simulink model "geothermal_simulink"  (R2024a)
settings: Solver=VariableStepAuto  StartTime=0.0  StopTime=10.0  RelTol=1e-3
libraries: spsStairGeneratorLib x1
settings Model: Creator=dogba  LastModifiedBy=dogba

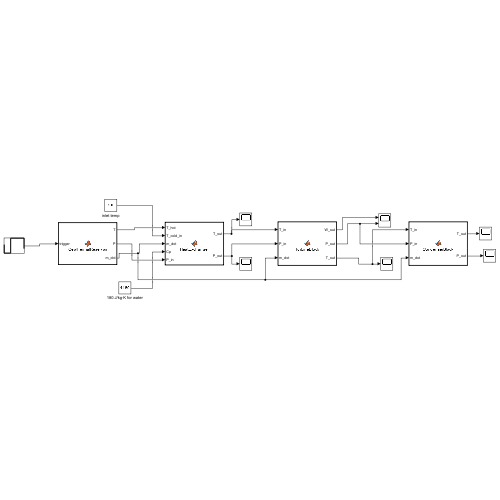
[thumbnail: Simulink's stored preview of the top-level diagram]
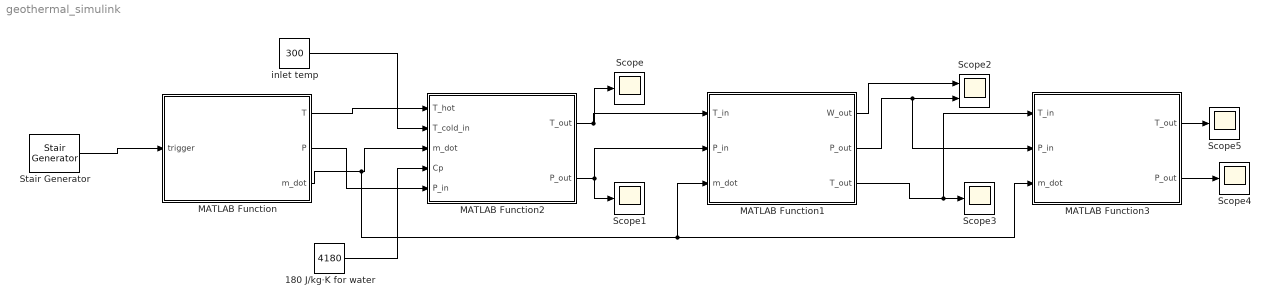
== system geothermal_simulink ==
  180 J/kg·K for water : Constant  Value=4180
  MATLAB Function : MATLAB Function  TreatAsAtomicUnit=on
  MATLAB Function1 : MATLAB Function  TreatAsAtomicUnit=on
  MATLAB Function2 : MATLAB Function  TreatAsAtomicUnit=on
  MATLAB Function3 : MATLAB Function  TreatAsAtomicUnit=on
  Scope{,1,3..5} (5 alike) : Scope
  Scope2 : Scope  NumInputPorts=2
  Stair Generator : spsStairGeneratorLib/Stair Generator  t=[0, 2,4, 8]  e=[1, -1, 2.5, 0]  Ts=0
  inlet temp : Constant  Value=300
  wires:
  MATLAB Function/2(P) -> MATLAB Function2/5(P_in)
  MATLAB Function/3(m_dot) -> MATLAB Function3/3(m_dot), MATLAB Function1/3(m_dot), MATLAB Function2/3(m_dot)
  MATLAB Function/1(T) -> MATLAB Function2/1(T_hot)
  180 J/kg·K for water/1 -> MATLAB Function2/4(Cp)
  inlet temp/1 -> MATLAB Function2/2(T_cold_in)
  MATLAB Function2/1(T_out) -> MATLAB Function1/1(T_in), Scope/1
  MATLAB Function2/2(P_out) -> Scope1/1, MATLAB Function1/2(P_in)
  MATLAB Function1/1(W_out) -> Scope2/1
  MATLAB Function1/2(P_out) -> MATLAB Function3/2(P_in), Scope2/2
  MATLAB Function1/3(T_out) -> MATLAB Function3/1(T_in), Scope3/1
  MATLAB Function3/2(P_out) -> Scope4/1
  MATLAB Function3/1(T_out) -> Scope5/1
  Stair Generator/1 -> MATLAB Function/1(trigger)

== matlab function geothermal_simulink/MATLAB Function1 ==
  data: W_out output; P_out output; T_in input; P_in input; T_out output; m_dot input
function [W_out, P_out, T_out] = TurbineBlock(T_in, P_in, m_dot)
% Custom turbine block
% Inputs:
%   T_in  - Inlet temperature (K)
%   P_in  - Inlet pressure (Pa)
%   m_dot - Mass flow rate (kg/s)
%
% Outputs:
%   W_out - Mechanical power output (W)
%   P_out - Outlet pressure (Pa)
%   T_out - Outlet temperature (K)

% Assumptions
efficiency = 0.75;        % Isentropic efficiency
P_out = 0.1e6;            % Low pressure (e.g., 0.1 MPa = 1 bar)
Cp = 4180;                % Specific heat of water (J/kg·K)
gamma = 1.33;             % For superheated steam (approximate)

% Isentropic temperature drop (ideal)
T_out_isentropic = T_in * (P_out / P_in)^((gamma - 1)/gamma);

% Real temperature drop
T_out = T_in - efficiency * (T_in - T_out_isentropic);

% Power output
W_out = m_dot * Cp * (T_in - T_out);   % Power (W)
end

== matlab function geothermal_simulink/MATLAB Function ==
  data: trigger input; T output; P output; m_dot output
function [T, P, m_dot] = GeothermalReservoir(trigger)
% Custom geothermal reservoir model

% Parameters
T = 473.15;         % Temperature in Kelvin (200°C)
P = 2e6;            % Pressure in Pascals
m_dot = 5;          % Mass flow rate (kg/s)

end

== matlab function geothermal_simulink/MATLAB Function2 ==
  data: T_hot input; T_out output; T_cold_in input; m_dot input; Cp input; P_in input; P_out output
function [T_out, P_out] = HeatExchanger(T_hot, T_cold_in, m_dot, Cp, P_in)
% Custom Heat Exchanger block
% Outputs:
%   T_out - Outlet temp of working fluid (K)
%   P_out - Outlet pressure (Pa)

epsilon = 0.85;
T_out = T_cold_in + epsilon * (T_hot - T_cold_in);

% Assume negligible pressure drop
P_out = P_in;
end

== matlab function geothermal_simulink/MATLAB Function3 ==
  data: T_out output; P_out output; T_in input; P_in input; m_dot input
function [T_out, P_out] = CondenserBlock(T_in, P_in, m_dot)
% Custom condenser block
% Inputs:
%   T_in  - Inlet temperature (K)
%   P_in  - Inlet pressure (Pa)
%   m_dot - Mass flow rate (kg/s)
%
% Outputs:
%   T_out - Outlet temperature (K)
%   P_out - Outlet pressure (Pa)

% Assumptions
T_cooling = 300;     % Cooling source temp (K)
efficiency = 0.9;    % Cooling efficiency
Cp = 4180;           % Water specific heat (J/kg.K)

% Simulate cooling
T_out = T_in - efficiency * (T_in - T_cooling);

% Assume small pressure drop or no change
P_out = P_in;
end
